simulink model "SpeedHold"  (R2022b)
settings: Solver=VariableStepAuto  StartTime=0.0  StopTime=100  RelTol=1e-3
undefined symbols (not defined in the file or in its folder): den_ut_p, num_ut_p
libraries: slpidlib x1
settings Model: Creator=^-^  LastModifiedBy=^-^

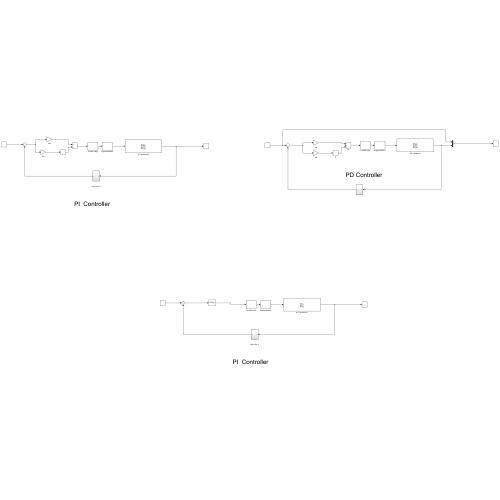
[thumbnail: Simulink's stored preview of the top-level diagram]
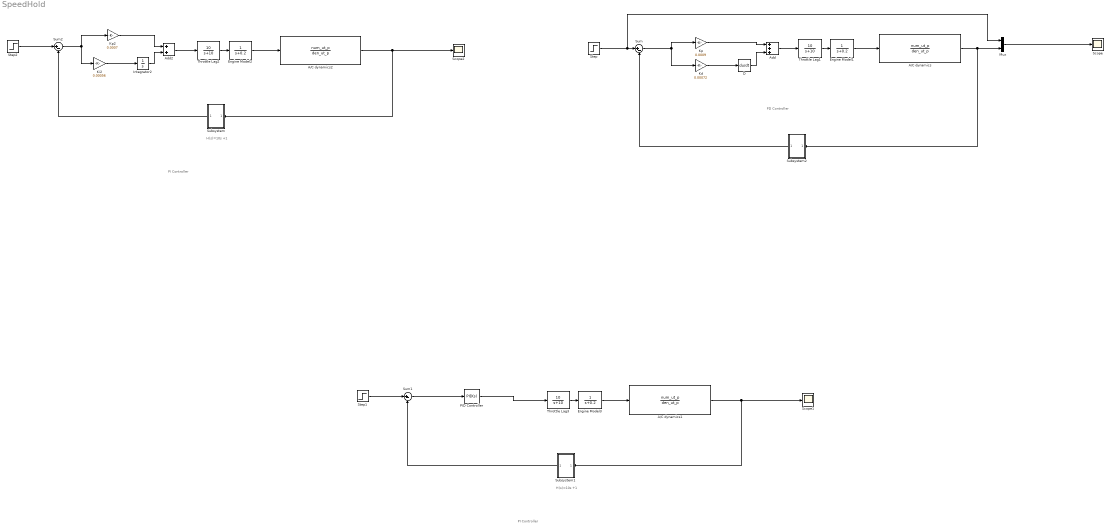
== system SpeedHold ==
  note: H(s)=10s +1
  note: PD Controller
  note: PI Controller
  note: H(s)=10s +1
  note: PI Controller
  A/C dynamics : TransferFcn  Numerator=num_ut_p  Denominator=den_ut_p
  A/C dynamics1 : TransferFcn  Numerator=num_ut_p  Denominator=den_ut_p
  A/C dynamics2 : TransferFcn  Numerator=num_ut_p  Denominator=den_ut_p
  Add : Sum  Inputs=+++
  Add2 : Sum
  D : Derivative
  Engine Model1 : TransferFcn  Numerator=1  Denominator=[1 0.2]
  Engine Model2 : TransferFcn  Numerator=1  Denominator=[1 0.2]
  Engine Model3 : TransferFcn  Numerator=1  Denominator=[1 0.2]
  Integrator2 : Integrator
  Kd : Gain  Gain=0.00072
  Ki2 : Gain  Gain=0.00056
  Kp : Gain  Gain=0.0009
  Kp2 : Gain  Gain=0.0007
  Mux : Mux  Inputs=2
  PID Controller : slpidlib/PID Controller  Controller=PID  Form=Parallel  TimeDomain=Continuous-time  UseExternalTs=off  SampleTime=-1  IntegratorMethod=Forward Euler  FilterMethod=Forward Euler  ControllerParametersSource=internal  P=0.0182799805611071  I=0.00130833442779242  UseKiTs=off  D=0.0502457069980119  N=5.66269492669485  UseFilter=on  TunerSelectOption=Transfer Function Based (PID Tuner App)  InitialConditionSource=internal  InitialConditionForIntegrator=0  InitialConditionForFilter=0  DifferentiatorICPrevScaledInput=0  ExternalReset=none  TrackingMode=off  Kt=1  LimitOutput=off  SatLimitsSource=internal  UpperSaturationLimit=inf  LowerSaturationLimit=-inf  LinearizeAsGain=on  AntiWindupMode=none  Kb=1  LimitIntegrator=off  UpperIntegratorSaturationLimit=inf  LowerIntegratorSaturationLimit=-inf  POutMin=[]  POutMax=[]  IOutMin=[]  IOutMax=[]  DOutMin=[]  DOutMax=[]  NOutMin=[]  NOutMax=[]  SumOutMin=[]  SumOutMax=[]  SaturationOutMin=[]  SaturationOutMax=[]  PParamMin=[]  PParamMax=[]  IParamMin=[]  IParamMax=[]  DParamMin=[]  DParamMax=[]  NParamMin=[]  NParamMax=[]  KbParamMin=[]  KbParamMax=[]  KtParamMin=[]  KtParamMax=[]  KbOutMin=[]  KbOutMax=[]  KtOutMin=[]  KtOutMax=[]  IntegratorOutMin=[]  IntegratorOutMax=[]  FilterOutMin=[]  FilterOutMax=[]  SumI1OutMin=[]  SumI1OutMax=[]  SumI2OutMin=[]  SumI2OutMax=[]  SumI3OutMin=[]  SumI3OutMax=[]  SumI4OutMin=[]  SumI4OutMax=[]  SumDOutMin=[]  SumDOutMax=[]  DifferentiatorOutMin=[]  DifferentiatorOutMax=[]  FilterDiffOutCoefMin=[]  FilterDiffOutCoefMax=[]  ReciprocalOutMin=[]  ReciprocalOutMax=[]  SumDenOutMin=[]  SumDenOutMax=[]  SumNumOutMin=[]  SumNumOutMax=[]  DivideOutMin=[]  DivideOutMax=[]  UdiffTsProdOutMin=[]  UdiffTsProdOutMax=[]  NTsProdOutMin=[]  NTsProdOutMax=[]  UintegralTsProdOutMin=[]  UintegralTsProdOutMax=[]  UngainTsProdOutMin=[]  UngainTsProdOutMax=[]  ClampingZeroOutDataTypeStr=Inherit: Inherit via back propagation  ClampingZeroOutMin=[]  ClampingZeroOutMax=[]  FilterDenConstantOutDataTypeStr=Inherit: Inherit via back propagation  FilterDenConstantOutMin=[]  FilterDenConstantOutMax=[]  PCopyOutDataTypeStr=Inherit: Inherit via back propagation  PCopyOutMin=[]  PCopyOutMax=[]  NCopyOutDataTypeStr=Inherit: Inherit via back propagation  NCopyOutMin=[]  NCopyOutMax=[]  IntegratorContinuousStateAttributes=''  IntegratorStateMustResolveToSignalObject=off  IntegratorRTWStateStorageClass=Auto  FilterContinuousStateAttributes=''  FilterStateMustResolveToSignalObject=off  FilterRTWStateStorageClass=Auto  ParallelPVariant=InternalParameters  IdealPVariant=Disabled  IVariant=InternalParameters  DVariant=InternalParameters  IntegratorVariant=Continuous  SatVariant=Disabled  AWVariant=Passthrough  PCopyVariant=Disabled  TRVariant=Disabled  FdbkBlocksVariant=Forward  IdealPFdbkVariant=Disabled  SatFdbkVariant=Disabled  DerivativeFilterVariant=ContFilter  NVariant=InternalParameters  NCopyVariant=Disabled  FilterICVariant=InternalICsFilter  IntegratorICVariant=InternalICs  ExternalResetVariant=Disabled  TRSumVariant=Passthrough  SumFdbkVariant=Disabled  SumVariant=Sum_PID  TsampFilterVariant=InternalTs  TsampNgainVariant=Passthrough  TsampIntegralVariant=Passthrough  ExternalSaturationOutDataTypeStr=Inherit: Same as second input
  Scope : Scope
  Scope1 : Scope
  Scope2 : Scope
  Step : Step  SampleTime=0
  Step1 : Step  SampleTime=0
  Step2 : Step  SampleTime=0
  Subsystem : Subsystem
  Subsystem1 : Subsystem
  Subsystem2 : Subsystem
  Sum : Sum  Inputs=|+-
  Sum1 : Sum  Inputs=|+-
  Sum2 : Sum  Inputs=|+-
  Throttle Lag1 : TransferFcn  Numerator=10  Denominator=[1 10]
  Throttle Lag2 : TransferFcn  Numerator=10  Denominator=[1 10]
  Throttle Lag3 : TransferFcn  Numerator=10  Denominator=[1 10]
  wires:
  Sum2/1 -> Ki2/1, Kp2/1
  Kp/1 -> Add/1
  Sum/1 -> Kp/1, Kd/1
  Mux/1 -> Scope/1
  Ki2/1 -> Integrator2/1
  Kd/1 -> D/1
  Integrator2/1 -> Add2/2
  Kp2/1 -> Add2/1
  A/C dynamics2/1 -> Scope2/1, Subsystem/1(In1)
  Step/1 -> Mux/1, Sum/1
  Step2/1 -> Sum2/1
  A/C dynamics/1 -> Subsystem2/1(In1), Mux/2
  D/1 -> Add/3
  Engine Model1/1 -> A/C dynamics/1
  Throttle Lag1/1 -> Engine Model1/1
  Add/1 -> Throttle Lag1/1
  Throttle Lag2/1 -> Engine Model2/1
  Add2/1 -> Throttle Lag2/1
  Engine Model2/1 -> A/C dynamics2/1
  Subsystem/1(Out1) -> Sum2/2
  Subsystem2/1(Out1) -> Sum/2
  Subsystem1/1(Out1) -> Sum1/2
  Throttle Lag3/1 -> Engine Model3/1
  Step1/1 -> Sum1/1
  A/C dynamics1/1 -> Scope1/1, Subsystem1/1(In1)
  Engine Model3/1 -> A/C dynamics1/1
  PID Controller/1 -> Throttle Lag3/1
  Sum1/1 -> PID Controller/1

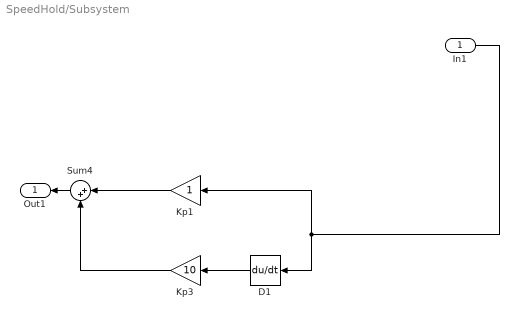
== system SpeedHold/Subsystem ==
  In1 : Inport
  D1 : Derivative
  Kp1 : Gain
  Kp3 : Gain  Gain=10
  Sum4 : Sum  Inputs=|++
  Out1 : Outport
  wires:
  In1/1 -> Kp1/1, D1/1
  D1/1 -> Kp3/1
  Kp3/1 -> Sum4/2
  Sum4/1 -> Out1/1
  Kp1/1 -> Sum4/1

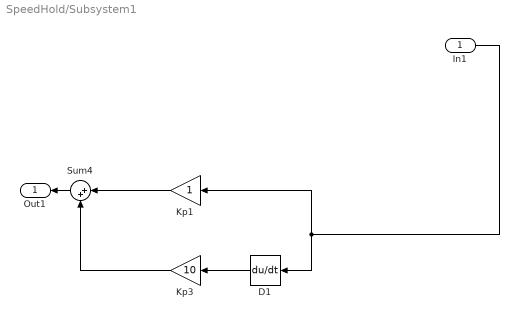
== system SpeedHold/Subsystem1 ==
  In1 : Inport
  D1 : Derivative
  Kp1 : Gain
  Kp3 : Gain  Gain=10
  Sum4 : Sum  Inputs=|++
  Out1 : Outport
  wires:
  In1/1 -> Kp1/1, D1/1
  D1/1 -> Kp3/1
  Kp3/1 -> Sum4/2
  Sum4/1 -> Out1/1
  Kp1/1 -> Sum4/1

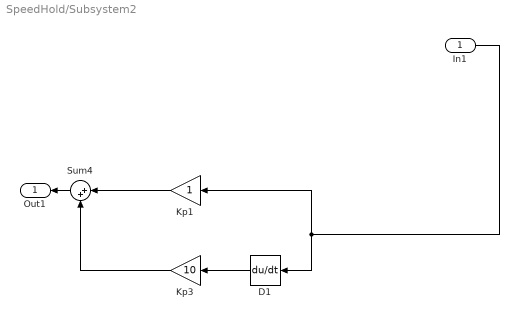
== system SpeedHold/Subsystem2 ==
  In1 : Inport
  D1 : Derivative
  Kp1 : Gain
  Kp3 : Gain  Gain=10
  Sum4 : Sum  Inputs=|++
  Out1 : Outport
  wires:
  In1/1 -> Kp1/1, D1/1
  D1/1 -> Kp3/1
  Kp3/1 -> Sum4/2
  Sum4/1 -> Out1/1
  Kp1/1 -> Sum4/1
